simulink model "regler_trottel_aterkoppling_img"  (R2012b)
settings: Solver=ode45  StartTime=0.0  StopTime=10.0  RelTol=1e-3
values from neighbouring files (symbols this model uses):
  KpThr = 1e-6    (= 1e-06)    [Init_Project2.m]
  TiThr = 0.1    [Init_Project2.m]
settings Model: Creator=rasme879  LastModifiedBy=rasme879

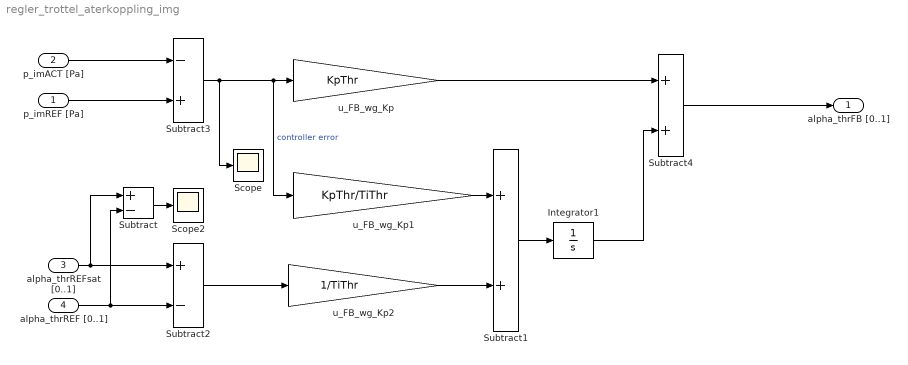
== system regler_trottel_aterkoppling_img ==
  p_imREF [Pa] : Inport
  p_imACT [Pa] : Inport  Port=2
  alpha_thrREFsat [0..1] : Inport  Port=3
  alpha_thrREF [0..1] : Inport  Port=4
  Integrator1 : Integrator  UpperSaturationLimit=5  LowerSaturationLimit=-5
  Scope : Scope
      settings: YMin=-110000  YMax=90000
  Scope2 : Scope
      settings: ShowLegends=on  YMin=-6  YMax=4.5
  Subtract : Sum  Inputs=+-
  Subtract1 : Sum
  Subtract2 : Sum  Inputs=+-
  Subtract3 : Sum  Inputs=-+
  Subtract4 : Sum
  u_FB_wg_Kp : Gain  Gain=KpThr
  u_FB_wg_Kp1 : Gain  Gain=KpThr/TiThr
  u_FB_wg_Kp2 : Gain  Gain=1/TiThr
  alpha_thrFB [0..1] : Outport
  wires:
  p_imACT [Pa]/1 -> Subtract3/1
  p_imREF [Pa]/1 -> Subtract3/2
  Subtract3/1 -> Scope/1, u_FB_wg_Kp/1, u_FB_wg_Kp1/1  "controller error"
  u_FB_wg_Kp/1 -> Subtract4/1
  Subtract4/1 -> alpha_thrFB [0..1]/1
  u_FB_wg_Kp1/1 -> Subtract1/1
  alpha_thrREFsat [0..1]/1 -> Subtract/1, Subtract2/1
  alpha_thrREF [0..1]/1 -> Subtract/2, Subtract2/2
  Subtract2/1 -> u_FB_wg_Kp2/1
  u_FB_wg_Kp2/1 -> Subtract1/2
  Subtract1/1 -> Integrator1/1
  Integrator1/1 -> Subtract4/2
  Subtract/1 -> Scope2/1
